simulink model "different_models"  (R2022a)
settings: Solver=ode23t  StartTime=0.0  StopTime=10  FixedStep=0.001  RelTol=1e-3
undefined symbols (not defined in the file or in its folder): Am, Bm, C_lqr_diff, Cm, Const_input, Dm, Kr, x_des
settings Model: Creator=asmax  LastModifiedBy=asmax
settings SolverCC: EnableFixedStepZeroCrossing=on

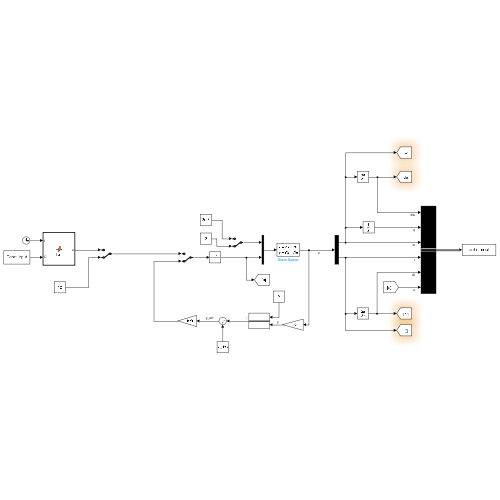
[thumbnail: Simulink's stored preview of the top-level diagram]
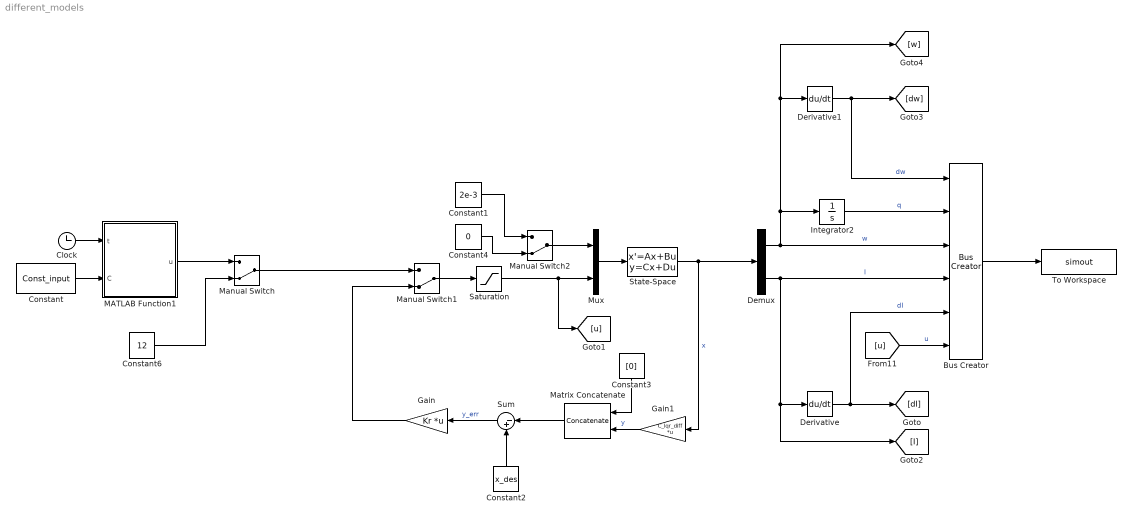
== system different_models ==
  Bus Creator : BusCreator  Inputs=6
  Clock : Clock
  Constant : Constant  Value=Const_input
  Constant1 : Constant  Value=2e-3
  Constant2 : Constant  Value=x_des
  Constant3 : Constant  Value=[0]
  Constant4 : Constant  Value=0
  Constant6 : Constant  Value=12
  Demux : Demux  Outputs=2
  Derivative : Derivative
  Derivative1 : Derivative
  Gain : Gain  Gain=Kr  Multiplication=Matrix(K*u)
  Gain1 : Gain  Gain=C_lqr_diff  Multiplication=Matrix(K*u)
  Integrator2 : Integrator
  MATLAB Function1 : MATLAB Function  TreatAsAtomicUnit=on
  Manual Switch : ManualSwitch  CurrentSetting=0
  Manual Switch1 : ManualSwitch  CurrentSetting=0
  Manual Switch2 : ManualSwitch  CurrentSetting=0
  Matrix Concatenate : Concatenate  ConcatenateDimension=2
  Mux : Mux  Inputs=2
  Saturation : Saturate  UpperLimit=15  LowerLimit=-15
  State-Space : StateSpace  A=Am  B=Bm  C=Cm  D=Dm  InitialCondition=[0;0]
  Sum : Sum  Inputs=|-+
  To Workspace : ToWorkspace  VariableName=simout  SaveFormat=Timeseries  SampleTime=-1
  wires:
  Mux/1 -> State-Space/1
  State-Space/1 -> Gain1/1, Demux/1  "x"
  Demux/1 -> Integrator2/1, [w], Derivative1/1, Bus Creator/3  "w"
  Demux/2 -> [I], Derivative/1, Bus Creator/4  "I"
  Bus Creator/1 -> To Workspace/1
  Derivative/1 -> Bus Creator/5, [dI]  "dI"
  Derivative1/1 -> [dw], Bus Creator/1  "dw"
  Clock/1 -> MATLAB Function1/1(t)
  MATLAB Function1/1(u) -> Manual Switch/1
  Constant6/1 -> Manual Switch/2
  Integrator2/1 -> Bus Creator/2  "q"
  [u] -> Bus Creator/6  "u"
  Constant/1 -> MATLAB Function1/2(C)
  Manual Switch/1 -> Manual Switch1/1
  Manual Switch1/1 -> Saturation/1
  Sum/1 -> Gain/1  "y_err"
  Constant2/1 -> Sum/2
  Gain/1 -> Manual Switch1/2
  Manual Switch2/1 -> Mux/1
  Constant1/1 -> Manual Switch2/1
  Gain1/1 -> Matrix Concatenate/2  "y"
  Matrix Concatenate/1 -> Sum/1
  Constant3/1 -> Matrix Concatenate/1
  Saturation/1 -> [u], Mux/2
  Constant4/1 -> Manual Switch2/2

== matlab function different_models/MATLAB Function1 ==
  data: t input; u output; C input
function u = fcn(t, C)

% w = 4;
% A = 6;
% B = 6;
% fi = 3.1415;
% u = A * cos(w * t + fi) + B;

w = C(3);
A = C(1);
B = C(2);
fi = C(4);
u = A * cos(w * t + fi) + B;
